simulink model "test3"  (R2020b)
settings: Solver=VariableStepAuto  StartTime=0.0  StopTime=10.0  RelTol=1e-3
settings Model: Creator=apple  LastModifiedBy=apple

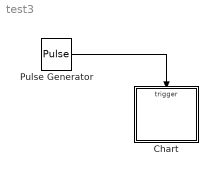
== system test3 ==
  Chart : Stateflow chart  TreatAsAtomicUnit=on
  Pulse Generator : DiscretePulseGenerator  PulseType=Time based  Period=1  PulseWidth=5
  wires:
  Pulse Generator/1 -> Chart/Trigger

== stateflow chart test3/Chart ==
  settings: sampleTime=1
  state A
    en:fprintf("enA");
    du:x=x+1;
    ex:fprintf("exA");
    on E: x = x + 1;
    state A1
    state A2
    (default) -> A1
    A1 -> A2 : {x=x+1;}
    A2 -> A1 : {x=x+1;}
    A -> A [order 1] : [x>1]{x=x+1;}
  (default) -> A : {x=0;}
  A -> A [order 1] : [x>3]{x=0;}
  data: x local
  events: E input EITHER_EDGE_EVENT
